simulink model "BallAndBeamControlado"  (R2018b)
settings: Solver=VariableStepAuto  StartTime=0.0  StopTime=ttotal  RelTol=1e-3
undefined symbols (not defined in the file or in its folder): ControlIncremental, p0, SimulBAB, tmuestra, Yr
settings Model: Creator=pablo  LastModifiedBy=pablo

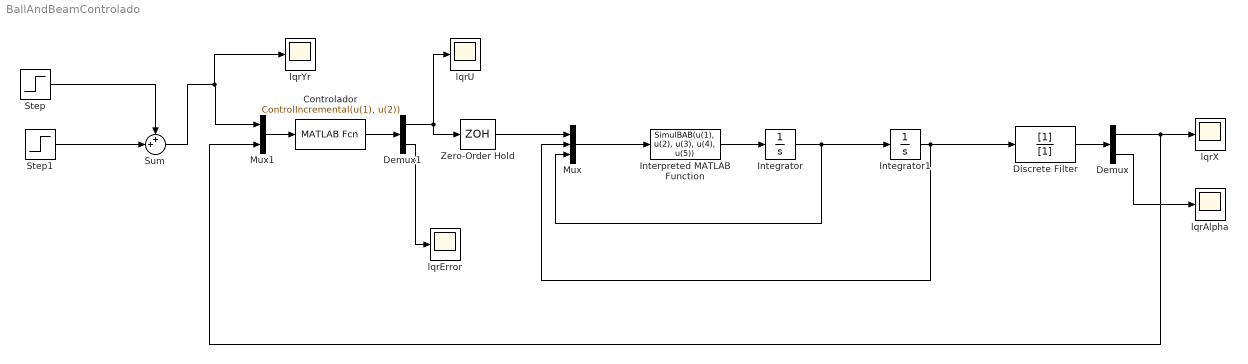
== system BallAndBeamControlado ==
  Controlador : MATLABFcn  MATLABFcn=ControlIncremental(u(1), u(2))  OutputDimensions=2
  Demux : Demux  Outputs=2
  Demux1 : Demux  Outputs=2
  Discrete Filter : DiscreteFilter  Denominator=[1]  SampleTime=tmuestra
  Integrator : Integrator  InitialCondition=[0 0]
  Integrator1 : Integrator  InitialCondition=[p0 0]
  Interpreted MATLAB Function : MATLABFcn  MATLABFcn=SimulBAB(u(1), u(2), u(3), u(4), u(5))  OutputDimensions=2
  Mux : Mux  Inputs=3
  Mux1 : Mux  Inputs=2
  Step : Step  After=Yr  SampleTime=tmuestra
  Step1 : Step  Time=5  After=-3*Yr  SampleTime=tmuestra
  Sum : Sum  Inputs=++|
  Zero-Order Hold : ZeroOrderHold  SampleTime=tmuestra
  "lqrAlpha " : Scope
  lqrError : Scope
  "lqrU " : Scope
  lqrX : Scope
  "lqrYr " : Scope
  wires:
  Mux/1 -> Interpreted MATLAB Function/1
  Zero-Order Hold/1 -> Mux/1
  Integrator/1 -> Integrator1/1, Mux/3
  Demux/2 -> "lqrAlpha "/1
  Demux/1 -> Mux1/2, lqrX/1
  Discrete Filter/1 -> Demux/1
  Mux1/1 -> Controlador/1
  Controlador/1 -> Demux1/1
  Demux1/1 -> "lqrU "/1, Zero-Order Hold/1
  Demux1/2 -> lqrError/1
  Interpreted MATLAB Function/1 -> Integrator/1
  Integrator1/1 -> Discrete Filter/1, Mux/2
  Sum/1 -> "lqrYr "/1, Mux1/1
  Step/1 -> Sum/1
  Step1/1 -> Sum/2
